simulink model "ExampleQueryTyre"  (Simulink 9.2)
settings: Solver=FixedStepDiscrete  StartTime=0.0  StopTime=inf  FixedStep=TIMESTEP  RelTol=1e-3  EnableMultiTasking=on
InitFcn:
  | TIMESTEP = 0.001;
libraries: rFproPhysicsLib x5
settings Model: Creator=marine  LastModifiedBy=SeanKavanagh
settings OptimizationCC: ExpressionDepthLimit=2147483647  InitFltsAndDblsToZero=on
settings DebuggingCC: SaveWithParameterizedLinksMsg=none  SolverPrmCheckMsg=warning
settings HardwareCC: TargetBitPerPointer=64  TargetBitPerSizeT=64  TargetBitPerPtrDiffT=64  TargetLongLongMode=on  TargetIntDivRoundTo=Zero  TargetEndianess=LittleEndian  TargetWordSize=64  TargetHWDeviceType=MATLAB Host  ProdEqTarget=off
settings RTWCC: SystemTargetFile=rsim.tlc  TemplateMakefile=rsim_default_tmf  Description=Rapid Simulation Target  TargetLang=C++
settings RSimTargetCC: PreserveStateflowLocalDataDimensions=off

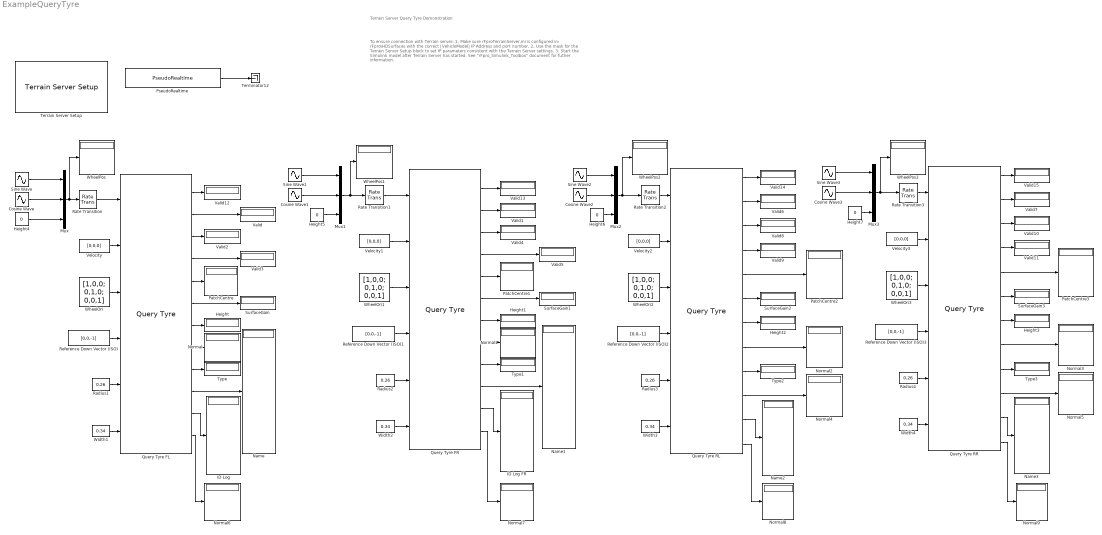
== system ExampleQueryTyre ==
  note: Terrain Server Query Tyre Demonstration
  note: To ensure connection with Terrain server:
      |
      | 1. Make sure rFproTerrainServer.ini is configured in: rFpro\HDSurfaces with the correct
      |     [VehicleModel] IP Address and port number.
      |
      | 2. Use the mask for the Terrain Server Setup block to set IP parameters consistent with
      |     the Terrain Server settings.
      |
      | 3. Start the Simulink model after Terrain Server has started.
      |
      | See "rFpro_Simulink_Toolbox" document for futher information.
  Cosine Wave{,1..3} (4 alike) : Sin  Amplitude=60  Bias=-620  Frequency=2*pi/20  Phase=pi/2  SampleTime=TIMESTEP
  Height{,1..3} (4 alike) : Display
  Height{4..7} (4 alike) : Constant  Value=0
  ID Log : Display
  ID Log FR : Display
  Mux{,1..3} (4 alike) : Mux  Inputs=3
  Name{,1..3} (4 alike) : Display
  Normal{,1..9} (10 alike) : Display
  PatchCentre{,1..3} (4 alike) : Display
  PseudoRealtime : S-Function  FunctionName=PseudoRealtime  Parameters=0.001  SFunctionDeploymentMode=off  EnableBusSupport=off
  Query Tyre FL : rFproPhysicsLib/Terrain Server Blocks/Query Tyre  wheel=FL  iso_mode=on  sampletime=0.001  phase_delay=0  roundtrip_frames=2  numUserDataElements=0  useReverseByteOrder=off  rFpro__TS_platform=Remote Model - Default  msgSize=0
  Query Tyre FR : rFproPhysicsLib/Terrain Server Blocks/Query Tyre  wheel=FR  iso_mode=on  sampletime=0.001  phase_delay=0  roundtrip_frames=2  numUserDataElements=0  useReverseByteOrder=off  rFpro__TS_platform=Remote Model - Default  msgSize=0
  Query Tyre RL : rFproPhysicsLib/Terrain Server Blocks/Query Tyre  wheel=RL  iso_mode=on  sampletime=0.001  phase_delay=0  roundtrip_frames=2  numUserDataElements=0  useReverseByteOrder=off  rFpro__TS_platform=Remote Model - Default  msgSize=0
  Query Tyre RR : rFproPhysicsLib/Terrain Server Blocks/Query Tyre  wheel=RR  iso_mode=on  sampletime=0.001  phase_delay=0  roundtrip_frames=2  numUserDataElements=0  useReverseByteOrder=off  rFpro__TS_platform=Remote Model - Default  msgSize=0
  Radius{1..4} (4 alike) : Constant  Value=0.26  OutDataTypeStr=double
  Rate Transition{,1..3} (4 alike) : RateTransition
  Reference Down Vector (ISO){,1..3} (4 alike) : Constant  Value=[0,0,-1]
  Sine Wave{,1..3} (4 alike) : Sin  Amplitude=60  Bias=821.6  Frequency=2*pi/20  SampleTime=TIMESTEP
  SurfaceGain{,1..3} (4 alike) : Display
  Terminator12 : Terminator
  Terrain Server Setup : rFproPhysicsLib/Terrain Server Blocks/Terrain Server Setup  Priority=0  track_name=''  tyre_config=[0.26, 0.34; 0.26, 0.34; 0.26, 0.34; 0.26, 0.34]  points_config="[0 1 0 0 0; 0 1  0.1125 0  0.05; 0 1  0.1125 0 -0.05; 0 1 -0.1125 0 -0.05; 0 1 -0.1125 0  0.05; 1 1  0      0  0; 1 1  0.1125 0  0.05; 1 1  0.1125 0 -0.05; 1 1 -0.1125 0 -0.05; 1 1 -0.1125 0  0.05; 2 1  0      0  0;  2 1  0.1125 0  0.05; 2 1  0.1125 0 -0.05; 2 1 -0.1125 0 -0.05; 2 1 -0.1125 0  0.05; 3 1  0      0  0; 3 1  0.1125 0  0.05; 3 1  0.1125 0 -0.05; 3 1 -0.1125 0 -0.05; 3 1 -0.1125 0  0.05]"  iso=on  triggerOnHeartbeat=off  heartbeat_latency=1750  rFpro__platform=Remote Model - Default  ts_address='127.0.0.1'  ts_port=11006  sendSampleTime=-1  sl_address='127.0.0.1'  sl_port=11002  receiveSampleTime=-1  maxUDPMsgs=8  useReverseByteOrder=off
  Type{,1..3} (4 alike) : Display
  Valid{,1..15} (16 alike) : Display
  Velocity{,1..3} (4 alike) : Constant  Value=[0,0,0]
  WheelOri{,1..3} (4 alike) : Constant  Value=[1,0,0; 0,1,0; 0,0,1]
  WheelPos{,1..3} (4 alike) : Display
  Width{1..4} (4 alike) : Constant  Value=0.34  OutDataTypeStr=double
  wires:
  WheelOri/1 -> Query Tyre FL/3
  Reference Down Vector (ISO)/1 -> Query Tyre FL/4
  Velocity/1 -> Query Tyre FL/2
  Mux1/1 -> WheelPos1/1, Rate Transition1/1
  WheelOri1/1 -> Query Tyre FR/3
  Reference Down Vector (ISO)1/1 -> Query Tyre FR/4
  Velocity1/1 -> Query Tyre FR/2
  Rate Transition2/1 -> Query Tyre RL/1
  WheelOri2/1 -> Query Tyre RL/3
  Reference Down Vector (ISO)2/1 -> Query Tyre RL/4
  Velocity2/1 -> Query Tyre RL/2
  Rate Transition3/1 -> Query Tyre RR/1
  WheelOri3/1 -> Query Tyre RR/3
  Reference Down Vector (ISO)3/1 -> Query Tyre RR/4
  Velocity3/1 -> Query Tyre RR/2
  Height4/1 -> Mux/3
  Mux/1 -> WheelPos/1, Rate Transition/1
  Sine Wave1/1 -> Mux1/1
  Cosine Wave1/1 -> Mux1/2
  Height5/1 -> Mux1/3
  Rate Transition/1 -> Query Tyre FL/1
  Rate Transition1/1 -> Query Tyre FR/1
  Query Tyre FR/1 -> Valid13/1
  Query Tyre FR/2 -> Valid1/1
  Query Tyre FR/3 -> Valid4/1
  Query Tyre FR/4 -> Valid5/1
  Query Tyre FR/5 -> PatchCentre1/1
  Query Tyre FR/7 -> Height1/1
  Query Tyre FL/1 -> Valid12/1
  Query Tyre FL/2 -> Valid/1
  Query Tyre FL/3 -> Valid2/1
  Query Tyre FL/4 -> Valid3/1
  Query Tyre FL/5 -> PatchCentre/1
  Query Tyre FL/6 -> SurfaceGain/1
  Query Tyre FL/7 -> Height/1
  Query Tyre FL/8 -> Normal/1
  Query Tyre FL/9 -> Type/1
  Query Tyre FL/11 -> ID Log/1
  Query Tyre FL/10 -> Name/1
  Query Tyre FR/6 -> SurfaceGain1/1
  Query Tyre FR/8 -> Normal1/1
  Query Tyre FR/9 -> Type1/1
  Query Tyre FR/10 -> Name1/1
  Query Tyre FR/11 -> ID Log FR/1
  Query Tyre RL/1 -> Valid14/1
  Query Tyre RL/2 -> Valid6/1
  Query Tyre RL/3 -> Valid8/1
  Query Tyre RL/4 -> Valid9/1
  Query Tyre RL/10 -> Normal4/1
  Query Tyre RL/11 -> Name2/1
  Query Tyre RL/5 -> PatchCentre2/1
  Query Tyre RL/6 -> SurfaceGain2/1
  Query Tyre RL/7 -> Height2/1
  Query Tyre RL/8 -> Normal2/1
  Query Tyre RL/9 -> Type2/1
  Query Tyre RR/1 -> Valid15/1
  Query Tyre RR/2 -> Valid7/1
  Query Tyre RR/3 -> Valid10/1
  Query Tyre RR/4 -> Valid11/1
  Query Tyre RR/5 -> PatchCentre3/1
  Query Tyre RR/6 -> SurfaceGain3/1
  Query Tyre RR/7 -> Height3/1
  Query Tyre RR/8 -> Normal3/1
  Query Tyre RR/9 -> Type3/1
  Query Tyre RR/10 -> Normal5/1
  Query Tyre RR/11 -> Name3/1
  PseudoRealtime/1 -> Terminator12/1
  Sine Wave/1 -> Mux/1
  Cosine Wave/1 -> Mux/2
  Mux2/1 -> WheelPos2/1, Rate Transition2/1
  Sine Wave2/1 -> Mux2/1
  Cosine Wave2/1 -> Mux2/2
  Height6/1 -> Mux2/3
  Mux3/1 -> WheelPos3/1, Rate Transition3/1
  Sine Wave3/1 -> Mux3/1
  Cosine Wave3/1 -> Mux3/2
  Height7/1 -> Mux3/3
  Radius1/1 -> Query Tyre FL/5
  Width1/1 -> Query Tyre FL/6
  Radius2/1 -> Query Tyre FR/5
  Width2/1 -> Query Tyre FR/6
  Radius3/1 -> Query Tyre RL/5
  Width3/1 -> Query Tyre RL/6
  Radius4/1 -> Query Tyre RR/5
  Width4/1 -> Query Tyre RR/6
  Query Tyre FL/12 -> Normal6/1
  Query Tyre FR/12 -> Normal7/1
  Query Tyre RL/12 -> Normal8/1
  Query Tyre RR/12 -> Normal9/1
